simulink model "seadrone_model"  (R2017a)
settings: Solver=VariableStepAuto  StartTime=0.0  StopTime=10.0  RelTol=1e-3
undefined symbols (not defined in the file): K, Tdelta, Tr
settings Model: Creator=Max  LastModifiedBy=Max

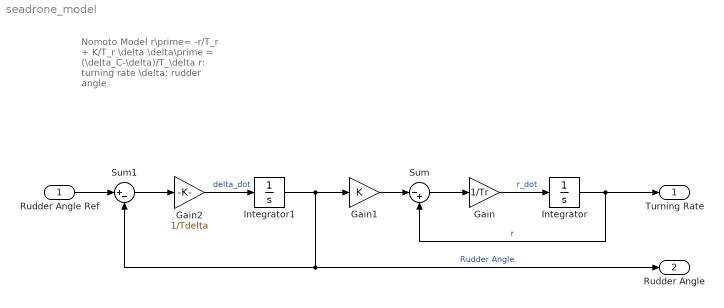
== system seadrone_model ==
  note: Nomoto Model
      |
      | r\prime= -r/T_r + K/T_r \delta
      | \delta\prime = (\delta_C-\delta)/T_\delta
      |
      | r: turning rate
      | \delta: rudder angle
  Rudder Angle Ref : Inport
  Gain : Gain  Gain=1/Tr
  Gain1 : Gain  Gain=K
  Gain2 : Gain  Gain=1/Tdelta
  Integrator : Integrator
  Integrator1 : Integrator
  Sum : Sum  Inputs=|-+
  Sum1 : Sum  Inputs=|+-
  Turning Rate : Outport
  Rudder Angle : Outport  Port=2
  wires:
  Gain/1 -> Integrator/1  "r_dot"
  Integrator/1 -> Turning Rate/1, Sum/2  "r"
  Gain2/1 -> Integrator1/1  "delta_dot"
  Integrator1/1 -> Rudder Angle/1, Sum1/2, Gain1/1  "Rudder Angle"
  Sum/1 -> Gain/1
  Gain1/1 -> Sum/1
  Sum1/1 -> Gain2/1
  Rudder Angle Ref/1 -> Sum1/1
